simulink model "carFollower"  (R2015b)
settings: Solver=VariableStepAuto  StartTime=0.0  StopTime=inf  FixedStep=0.1  RelTol=1e-3
undefined symbols (not defined in the file or in its folder): Angular, Linear
libraries: robotlib x6, fuzblock x1
settings Model: Creator=sprinkle  LastModifiedBy=sprinkle

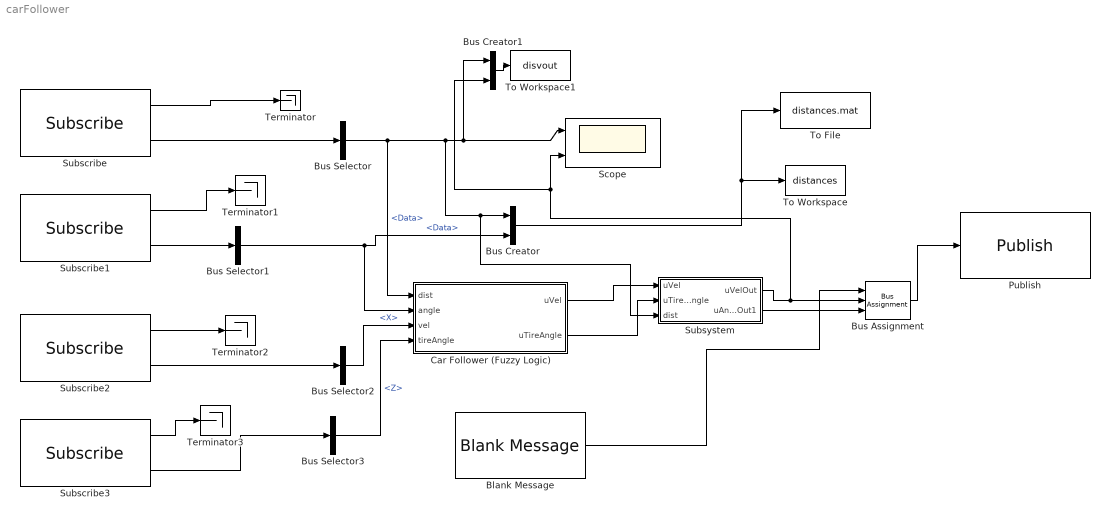
== system carFollower ==
  Blank Message : robotlib/Blank Message  SourceLibraryInfo=This block requires Robotics System Toolbox  messageType=geometry_msgs/Twist  SampleTime=inf
  Bus Assignment : BusAssignment  AssignedSignals=Linear.X,Angular.Z
  Bus Creator : BusCreator  Inputs=2
  Bus Creator1 : BusCreator  Inputs=2
  Bus Selector : BusSelector  OutputSignals=Data
  Bus Selector1 : BusSelector  OutputSignals=Data
  Bus Selector2 : BusSelector  OutputSignals=Linear.X
  Bus Selector3 : BusSelector  OutputSignals=Torque.Z
  Car Follower (Fuzzy Logic) : Subsystem  TreatAsAtomicUnit=on
  Publish : robotlib/Publish  SourceLibraryInfo=This block requires Robotics System Toolbox  topicSource=Select from ROS network  topic=/follower_sim/cmd_vel  messageType=geometry_msgs/Twist  messageQueueLength=1
  Scope : Scope  NumInputPorts=2
  Subscribe : robotlib/Subscribe  SourceLibraryInfo=This block requires Robotics System Toolbox  topicSource=Select from ROS network  topic=/follower_sim/distanceEstimator/dist  messageType=std_msgs/Float32  sampleTime=-1  messageQueueLength=1
  Subscribe1 : robotlib/Subscribe  SourceLibraryInfo=This block requires Robotics System Toolbox  topicSource=Select from ROS network  topic=/follower_sim/distanceEstimator/angle  messageType=std_msgs/Float32  sampleTime=-1  messageQueueLength=1
  Subscribe2 : robotlib/Subscribe  SourceLibraryInfo=This block requires Robotics System Toolbox  topicSource=Select from ROS network  topic=/follower_sim/vel  messageType=geometry_msgs/Twist  sampleTime=-1  messageQueueLength=1
  Subscribe3 : robotlib/Subscribe  SourceLibraryInfo=This block requires Robotics System Toolbox  topicSource=Select from ROS network  topic=/follower_sim/steering  messageType=geometry_msgs/Wrench  sampleTime=-1  messageQueueLength=1
  Subsystem : Subsystem
  Terminator{,1..3} (4 alike) : Terminator
  To File : ToFile  Filename=distances.mat  MatrixName=DistanceEstimator  SaveFormat=Timeseries
  To Workspace : ToWorkspace  VariableName=distances  SaveFormat=Timeseries  SampleTime=-1
  To Workspace1 : ToWorkspace  VariableName=disvout  SaveFormat=Timeseries  SampleTime=-1
  wires:
  Subscribe/2 -> Bus Selector/1
  Subscribe/1 -> Terminator/1
  Subscribe1/2 -> Bus Selector1/1
  Bus Assignment/1 -> Publish/1
  Subscribe1/1 -> Terminator1/1
  Blank Message/1 -> Bus Assignment/1
  Bus Selector/1 -> Car Follower (Fuzzy Logic)/1(dist), Bus Creator1/1, Scope/1, Subsystem/3(dist), Bus Creator/1  "<Data>"
  Bus Selector1/1 -> Car Follower (Fuzzy Logic)/2(angle), Bus Creator/2  "<Data>"
  Bus Creator/1 -> To File/1, To Workspace/1
  Subscribe2/1 -> Terminator2/1
  Subscribe2/2 -> Bus Selector2/1
  Subscribe3/2 -> Bus Selector3/1
  Bus Selector3/1 -> Car Follower (Fuzzy Logic)/4(tireAngle)  "<Z>"
  Bus Selector2/1 -> Car Follower (Fuzzy Logic)/3(vel)  "<X>"
  Subscribe3/1 -> Terminator3/1
  Car Follower (Fuzzy Logic)/1(uVel) -> Subsystem/1(uVel)
  Car Follower (Fuzzy Logic)/2(uTireAngle) -> Subsystem/2(uTireAngle)
  Subsystem/1(uVelOut) -> Bus Creator1/2, Scope/2, Bus Assignment/2
  Subsystem/2(uAngleOut1) -> Bus Assignment/3
  Bus Creator1/1 -> To Workspace1/1

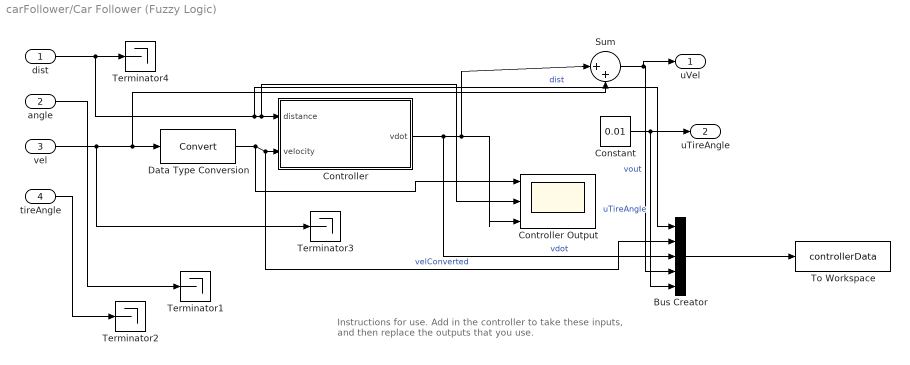
== system carFollower/Car Follower (Fuzzy Logic) ==
  note: Instructions for use.
      |
      | Add in the controller to take these inputs, and then replace
      | the outputs that you use.
  dist : Inport
  angle : Inport  Port=2
  vel : Inport  Port=3
  tireAngle : Inport  Port=4
  Bus Creator : BusCreator  Inputs=5
  Constant : Constant  Value=0.01
  Controller : Subsystem
  Controller Output : Scope  NumInputPorts=3
  Data Type Conversion : DataTypeConversion  RndMeth=Nearest
  Sum : Sum  Inputs=|++
  Terminator{1..4} (4 alike) : Terminator
  To Workspace : ToWorkspace  VariableName=controllerData  SaveFormat=Timeseries  SampleTime=-1
  uVel : Outport
  uTireAngle : Outport  Port=2
  wires:
  Sum/1 -> Bus Creator/4, uVel/1  "vout"
  tireAngle/1 -> Terminator2/1
  angle/1 -> Terminator1/1
  Constant/1 -> Bus Creator/5, uTireAngle/1  "uTireAngle"
  vel/1 -> Sum/2, Data Type Conversion/1, Terminator3/1
  dist/1 -> Bus Creator/1, Controller Output/2, Controller/1(distance), Terminator4/1  "dist"
  Controller/1(vdot) -> Bus Creator/3, Sum/1, Controller Output/3  "vdot"
  Data Type Conversion/1 -> Controller Output/1, Bus Creator/2, Controller/2(velocity)  "velConverted"
  Bus Creator/1 -> To Workspace/1

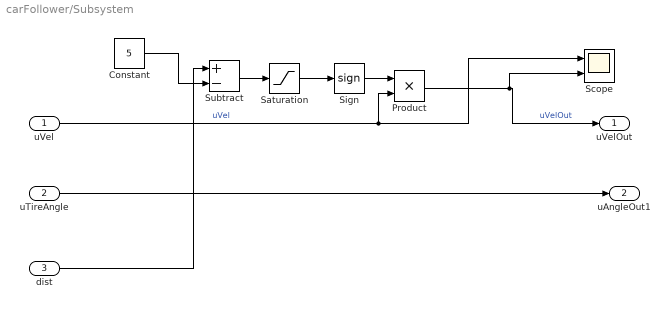
== system carFollower/Subsystem ==
  uVel : Inport
  uTireAngle : Inport  Port=2
  dist : Inport  Port=3
  Constant : Constant  Value=5
  Product : Product
  Saturation : Saturate  UpperLimit=1  LowerLimit=0
  Scope : Scope  NumInputPorts=2
  Sign : Signum
  Subtract : Sum  Inputs=+-
  uVelOut : Outport
  uAngleOut1 : Outport  Port=2
  wires:
  Constant/1 -> Subtract/2
  dist/1 -> Subtract/1
  Subtract/1 -> Saturation/1
  Saturation/1 -> Sign/1
  uVel/1 -> Scope/1, Product/2  "uVel"
  Sign/1 -> Product/1
  Product/1 -> Scope/2, uVelOut/1  "uVelOut"
  uTireAngle/1 -> uAngleOut1/1

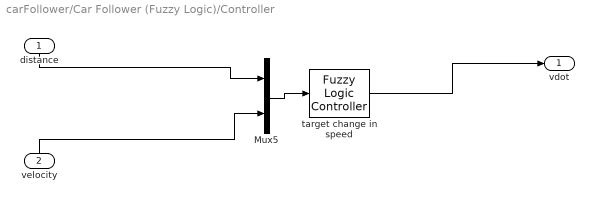
== system carFollower/Car Follower (Fuzzy Logic)/Controller ==
  distance : Inport
  velocity : Inport  Port=2
  Mux5 : Mux  Inputs=2
  target change in speed : fuzblock/Fuzzy Logic  Controller  fis='spring2.fis'
  vdot : Outport
  wires:
  distance/1 -> Mux5/1
  velocity/1 -> Mux5/2
  Mux5/1 -> target change in speed/1
  target change in speed/1 -> vdot/1
